simulink model "Planner"  (R2019a)
settings: Solver=FixedStepAuto  StartTime=0.0  StopTime=10.0  FixedStep=0.001  RelTol=1e-3
settings Model: Creator=EiLit  LastModifiedBy=EiLit
settings DataIOCC: ReturnWorkspaceOutputs=off
settings DebuggingCC: ArithmeticOperatorsInVariantConditions=warning

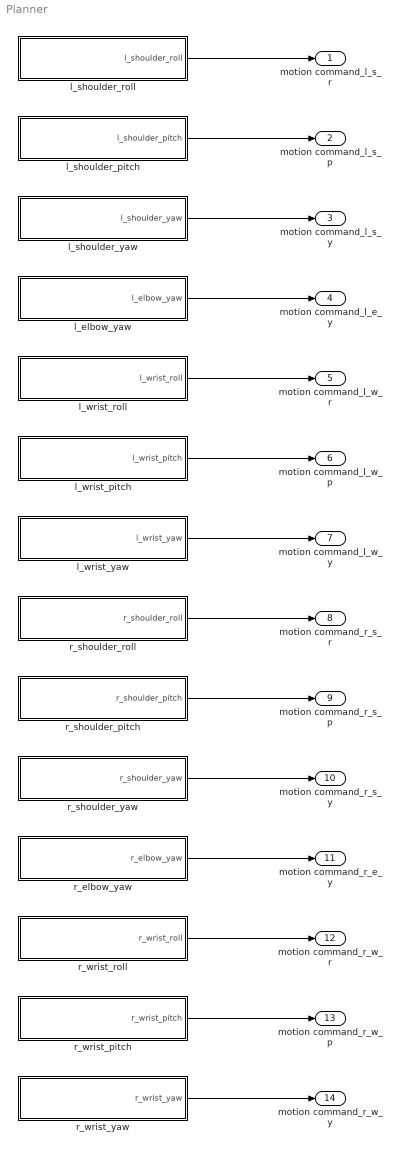
== system Planner ==
  l_elbow_yaw : Subsystem
  l_shoulder_pitch : Subsystem
  l_shoulder_roll : Subsystem
  l_shoulder_yaw : Subsystem
  l_wrist_pitch : Subsystem
  l_wrist_roll : Subsystem
  l_wrist_yaw : Subsystem
  r_elbow_yaw : Subsystem
  r_shoulder_pitch : Subsystem
  r_shoulder_roll : Subsystem
  r_shoulder_yaw : Subsystem
  r_wrist_pitch : Subsystem
  r_wrist_roll : Subsystem
  r_wrist_yaw : Subsystem
  motion command_l_s_r : Outport
  motion command_l_s_p : Outport  Port=2
  motion command_l_s_y : Outport  Port=3
  motion command_l_e_y : Outport  Port=4
  motion command_l_w_r : Outport  Port=5
  motion command_l_w_p : Outport  Port=6
  motion command_l_w_y : Outport  Port=7
  motion command_r_s_r : Outport  Port=8
  motion command_r_s_p : Outport  Port=9
  motion command_r_s_y : Outport  Port=10
  motion command_r_e_y : Outport  Port=11
  motion command_r_w_r : Outport  Port=12
  motion command_r_w_p : Outport  Port=13
  motion command_r_w_y : Outport  Port=14
  wires:
  r_shoulder_yaw/1(r_shoulder_yaw) -> motion command_r_s_y/1
  l_wrist_yaw/1(l_wrist_yaw) -> motion command_l_w_y/1
  l_elbow_yaw/1(l_elbow_yaw) -> motion command_l_e_y/1
  l_shoulder_yaw/1(l_shoulder_yaw) -> motion command_l_s_y/1
  r_elbow_yaw/1(r_elbow_yaw) -> motion command_r_e_y/1
  l_wrist_pitch/1(l_wrist_pitch) -> motion command_l_w_p/1
  l_shoulder_roll/1(l_shoulder_roll) -> motion command_l_s_r/1
  r_wrist_pitch/1(r_wrist_pitch) -> motion command_r_w_p/1
  l_wrist_roll/1(l_wrist_roll) -> motion command_l_w_r/1
  r_shoulder_pitch/1(r_shoulder_pitch) -> motion command_r_s_p/1
  l_shoulder_pitch/1(l_shoulder_pitch) -> motion command_l_s_p/1
  r_wrist_yaw/1(r_wrist_yaw) -> motion command_r_w_y/1
  r_shoulder_roll/1(r_shoulder_roll) -> motion command_r_s_r/1
  r_wrist_roll/1(r_wrist_roll) -> motion command_r_w_r/1

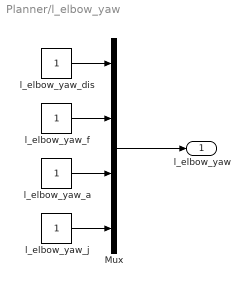
== system Planner/l_elbow_yaw ==
  Mux : Mux
  l_elbow_yaw_a : Constant
  l_elbow_yaw_dis : Constant
  l_elbow_yaw_f : Constant
  l_elbow_yaw_j : Constant
  l_elbow_yaw : Outport
  wires:
  l_elbow_yaw_dis/1 -> Mux/1
  l_elbow_yaw_f/1 -> Mux/2
  Mux/1 -> l_elbow_yaw/1
  l_elbow_yaw_a/1 -> Mux/3
  l_elbow_yaw_j/1 -> Mux/4

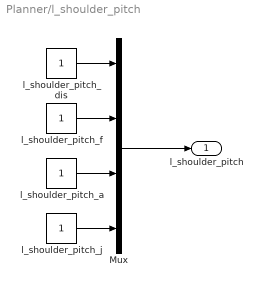
== system Planner/l_shoulder_pitch ==
  Mux : Mux
  l_shoulder_pitch_a : Constant
  l_shoulder_pitch_dis : Constant
  l_shoulder_pitch_f : Constant
  l_shoulder_pitch_j : Constant
  l_shoulder_pitch : Outport
  wires:
  l_shoulder_pitch_dis/1 -> Mux/1
  l_shoulder_pitch_f/1 -> Mux/2
  Mux/1 -> l_shoulder_pitch/1
  l_shoulder_pitch_a/1 -> Mux/3
  l_shoulder_pitch_j/1 -> Mux/4

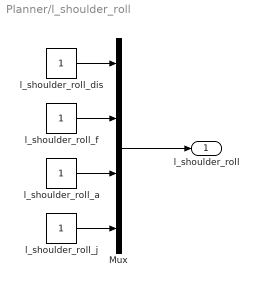
== system Planner/l_shoulder_roll ==
  Mux : Mux
  l_shoulder_roll_a : Constant
  l_shoulder_roll_dis : Constant
  l_shoulder_roll_f : Constant
  l_shoulder_roll_j : Constant
  l_shoulder_roll : Outport
  wires:
  l_shoulder_roll_j/1 -> Mux/4
  l_shoulder_roll_a/1 -> Mux/3
  Mux/1 -> l_shoulder_roll/1
  l_shoulder_roll_f/1 -> Mux/2
  l_shoulder_roll_dis/1 -> Mux/1

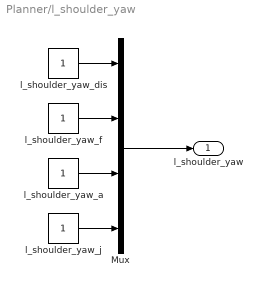
== system Planner/l_shoulder_yaw ==
  Mux : Mux
  l_shoulder_yaw_a : Constant
  l_shoulder_yaw_dis : Constant
  l_shoulder_yaw_f : Constant
  l_shoulder_yaw_j : Constant
  l_shoulder_yaw : Outport
  wires:
  l_shoulder_yaw_j/1 -> Mux/4
  l_shoulder_yaw_a/1 -> Mux/3
  Mux/1 -> l_shoulder_yaw/1
  l_shoulder_yaw_f/1 -> Mux/2
  l_shoulder_yaw_dis/1 -> Mux/1

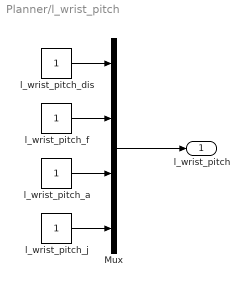
== system Planner/l_wrist_pitch ==
  Mux : Mux
  l_wrist_pitch_a : Constant
  l_wrist_pitch_dis : Constant
  l_wrist_pitch_f : Constant
  l_wrist_pitch_j : Constant
  l_wrist_pitch : Outport
  wires:
  l_wrist_pitch_dis/1 -> Mux/1
  l_wrist_pitch_f/1 -> Mux/2
  Mux/1 -> l_wrist_pitch/1
  l_wrist_pitch_a/1 -> Mux/3
  l_wrist_pitch_j/1 -> Mux/4

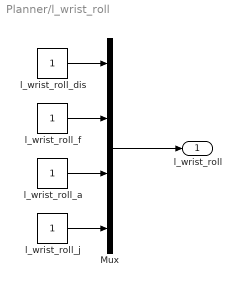
== system Planner/l_wrist_roll ==
  Mux : Mux
  l_wrist_roll_a : Constant
  l_wrist_roll_dis : Constant
  l_wrist_roll_f : Constant
  l_wrist_roll_j : Constant
  l_wrist_roll : Outport
  wires:
  l_wrist_roll_j/1 -> Mux/4
  l_wrist_roll_a/1 -> Mux/3
  Mux/1 -> l_wrist_roll/1
  l_wrist_roll_f/1 -> Mux/2
  l_wrist_roll_dis/1 -> Mux/1

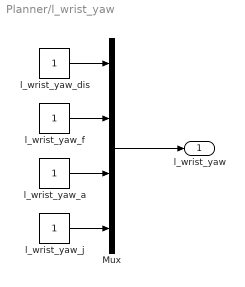
== system Planner/l_wrist_yaw ==
  Mux : Mux
  l_wrist_yaw_a : Constant
  l_wrist_yaw_dis : Constant
  l_wrist_yaw_f : Constant
  l_wrist_yaw_j : Constant
  l_wrist_yaw : Outport
  wires:
  l_wrist_yaw_j/1 -> Mux/4
  l_wrist_yaw_a/1 -> Mux/3
  Mux/1 -> l_wrist_yaw/1
  l_wrist_yaw_f/1 -> Mux/2
  l_wrist_yaw_dis/1 -> Mux/1

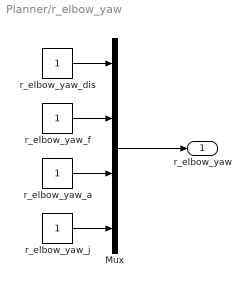
== system Planner/r_elbow_yaw ==
  Mux : Mux
  r_elbow_yaw_a : Constant
  r_elbow_yaw_dis : Constant
  r_elbow_yaw_f : Constant
  r_elbow_yaw_j : Constant
  r_elbow_yaw : Outport
  wires:
  r_elbow_yaw_j/1 -> Mux/4
  r_elbow_yaw_a/1 -> Mux/3
  Mux/1 -> r_elbow_yaw/1
  r_elbow_yaw_f/1 -> Mux/2
  r_elbow_yaw_dis/1 -> Mux/1

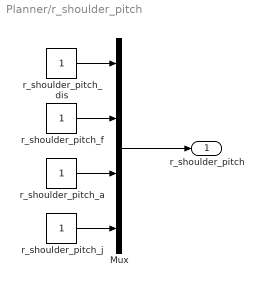
== system Planner/r_shoulder_pitch ==
  Mux : Mux
  r_shoulder_pitch_a : Constant
  r_shoulder_pitch_dis : Constant
  r_shoulder_pitch_f : Constant
  r_shoulder_pitch_j : Constant
  r_shoulder_pitch : Outport
  wires:
  r_shoulder_pitch_j/1 -> Mux/4
  r_shoulder_pitch_a/1 -> Mux/3
  Mux/1 -> r_shoulder_pitch/1
  r_shoulder_pitch_f/1 -> Mux/2
  r_shoulder_pitch_dis/1 -> Mux/1

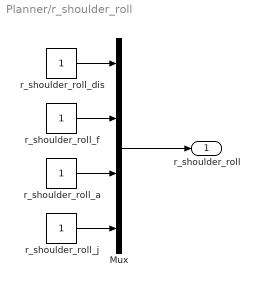
== system Planner/r_shoulder_roll ==
  Mux : Mux
  r_shoulder_roll_a : Constant
  r_shoulder_roll_dis : Constant
  r_shoulder_roll_f : Constant
  r_shoulder_roll_j : Constant
  r_shoulder_roll : Outport
  wires:
  r_shoulder_roll_dis/1 -> Mux/1
  r_shoulder_roll_f/1 -> Mux/2
  Mux/1 -> r_shoulder_roll/1
  r_shoulder_roll_a/1 -> Mux/3
  r_shoulder_roll_j/1 -> Mux/4

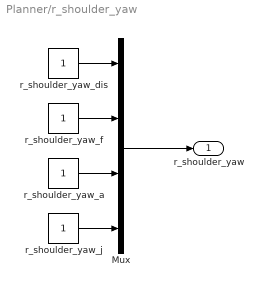
== system Planner/r_shoulder_yaw ==
  Mux : Mux
  r_shoulder_yaw_a : Constant
  r_shoulder_yaw_dis : Constant
  r_shoulder_yaw_f : Constant
  r_shoulder_yaw_j : Constant
  r_shoulder_yaw : Outport
  wires:
  r_shoulder_yaw_dis/1 -> Mux/1
  r_shoulder_yaw_f/1 -> Mux/2
  Mux/1 -> r_shoulder_yaw/1
  r_shoulder_yaw_a/1 -> Mux/3
  r_shoulder_yaw_j/1 -> Mux/4

== system Planner/r_wrist_pitch ==
  Mux : Mux
  r_wrist_pitch_a : Constant
  r_wrist_pitch_dis : Constant
  r_wrist_pitch_f : Constant
  r_wrist_pitch_j : Constant
  r_wrist_pitch : Outport
  wires:
  r_wrist_pitch_j/1 -> Mux/4
  r_wrist_pitch_a/1 -> Mux/3
  Mux/1 -> r_wrist_pitch/1
  r_wrist_pitch_f/1 -> Mux/2
  r_wrist_pitch_dis/1 -> Mux/1

== system Planner/r_wrist_roll ==
  Mux : Mux
  r_wrist_roll_a : Constant
  r_wrist_roll_dis : Constant
  r_wrist_roll_f : Constant
  r_wrist_roll_j : Constant
  r_wrist_roll : Outport
  wires:
  r_wrist_roll_dis/1 -> Mux/1
  r_wrist_roll_f/1 -> Mux/2
  Mux/1 -> r_wrist_roll/1
  r_wrist_roll_a/1 -> Mux/3
  r_wrist_roll_j/1 -> Mux/4

== system Planner/r_wrist_yaw ==
  Mux : Mux
  r_wrist_yaw_a : Constant
  r_wrist_yaw_dis : Constant
  r_wrist_yaw_f : Constant
  r_wrist_yaw_j : Constant
  r_wrist_yaw : Outport
  wires:
  r_wrist_yaw_dis/1 -> Mux/1
  r_wrist_yaw_f/1 -> Mux/2
  Mux/1 -> r_wrist_yaw/1
  r_wrist_yaw_a/1 -> Mux/3
  r_wrist_yaw_j/1 -> Mux/4
